simulink model "gm_inc_enc_v26_vnl"  (R2023a)
settings: Solver=FixedStepDiscrete  StartTime=0.0  StopTime=SimulationsDauer  RelTol=1e-3
undefined symbols (not defined in the file or in its folder): CW_CCW_Switch, d_axis_hit_CompareValue, DiscIntNeverNeededParam, f_ISR, IncPerTurn, inital_zero_speed_timeout, n_max, Offset_Position_elec, Offset_Position_mech, OmegaPerOverSampl, Periode, Phase_Delay_A, Phase_Delay_B, PolePair, QuadratureFactor, reciprocal_iterations, T_fpga, T_mech
libraries: simulink x25, hdlmdlgenlib x16, hdlsllib x4, dspsrcs4 x3, dspswit3 x2, spsEdgeDetectorLib x2, simulink_extras x1
(part 2 of 5)

== system gm_inc_enc_v26_vnl/Compare/Assert_count ==
  cosim : Inport
  dut : Inport  Port=2
  AssertEq : Assertion  StopWhenAssertionFail=off
  Compare To Zero : simulink/Logic and Bit Operations/Compare To Zero  relop===  OutDataTypeStr=boolean
  Relational Operator : RelationalOperator  Operator===  OutDataTypeStr=boolean  InputSameDT=off
  compare: count : Scope  NumInputPorts=3
  wires:
  Compare To Zero/1 -> compare: count/3  "err"
  Relational Operator/1 -> Compare To Zero/1, AssertEq/1
  cosim/1 -> compare: count/1, Relational Operator/1  "cosim"
  dut/1 -> compare: count/2, Relational Operator/2  "dut ref"

== system gm_inc_enc_v26_vnl/Compare/Assert_countPerPeriod_AXI4 ==
  cosim : Inport
  dut : Inport  Port=2
  AssertEq : Assertion  StopWhenAssertionFail=off
  Compare To Zero : simulink/Logic and Bit Operations/Compare To Zero  relop===  OutDataTypeStr=boolean
  Relational Operator : RelationalOperator  Operator===  OutDataTypeStr=boolean  InputSameDT=off
  compare: countPerPeriod_AXI4 : Scope  NumInputPorts=3
  wires:
  Compare To Zero/1 -> compare: countPerPeriod_AXI4/3  "err"
  Relational Operator/1 -> Compare To Zero/1, AssertEq/1
  cosim/1 -> compare: countPerPeriod_AXI4/1, Relational Operator/1  "cosim"
  dut/1 -> compare: countPerPeriod_AXI4/2, Relational Operator/2  "dut ref"

== system gm_inc_enc_v26_vnl/Compare/Assert_d-Axis-Hit ==
  cosim : Inport
  dut : Inport  Port=2
  AssertEq : Assertion  StopWhenAssertionFail=off
  Compare To Zero : simulink/Logic and Bit Operations/Compare To Zero  relop===  OutDataTypeStr=boolean
  Relational Operator : RelationalOperator  Operator===  OutDataTypeStr=boolean  InputSameDT=off
  compare: d-Axis-Hit : Scope  NumInputPorts=3
  wires:
  Compare To Zero/1 -> compare: d-Axis-Hit/3  "err"
  Relational Operator/1 -> Compare To Zero/1, AssertEq/1
  cosim/1 -> compare: d-Axis-Hit/1, Relational Operator/1  "cosim"
  dut/1 -> compare: d-Axis-Hit/2, Relational Operator/2  "dut ref"

== system gm_inc_enc_v26_vnl/Compare/Assert_d-Axis-Hit_WithCompare ==
  cosim : Inport
  dut : Inport  Port=2
  AssertEq : Assertion  StopWhenAssertionFail=off
  Compare To Zero : simulink/Logic and Bit Operations/Compare To Zero  relop===  OutDataTypeStr=boolean
  Relational Operator : RelationalOperator  Operator===  OutDataTypeStr=boolean  InputSameDT=off
  compare: d-Axis-Hit_WithCompare : Scope  NumInputPorts=3
  wires:
  Compare To Zero/1 -> compare: d-Axis-Hit_WithCompare/3  "err"
  Relational Operator/1 -> Compare To Zero/1, AssertEq/1
  cosim/1 -> compare: d-Axis-Hit_WithCompare/1, Relational Operator/1  "cosim"
  dut/1 -> compare: d-Axis-Hit_WithCompare/2, Relational Operator/2  "dut ref"

== system gm_inc_enc_v26_vnl/Compare/Assert_direction_AXI4 ==
  cosim : Inport
  dut : Inport  Port=2
  AssertEq : Assertion  StopWhenAssertionFail=off
  Compare To Zero : simulink/Logic and Bit Operations/Compare To Zero  relop===  OutDataTypeStr=boolean
  Relational Operator : RelationalOperator  Operator===  OutDataTypeStr=boolean  InputSameDT=off
  compare: direction_AXI4 : Scope  NumInputPorts=3
  wires:
  Compare To Zero/1 -> compare: direction_AXI4/3  "err"
  Relational Operator/1 -> Compare To Zero/1, AssertEq/1
  cosim/1 -> compare: direction_AXI4/1, Relational Operator/1  "cosim"
  dut/1 -> compare: direction_AXI4/2, Relational Operator/2  "dut ref"

== system gm_inc_enc_v26_vnl/Compare/Assert_edge ==
  cosim : Inport
  dut : Inport  Port=2
  AssertEq : Assertion  StopWhenAssertionFail=off
  Compare To Zero : simulink/Logic and Bit Operations/Compare To Zero  relop===  OutDataTypeStr=boolean
  Relational Operator : RelationalOperator  Operator===  OutDataTypeStr=boolean  InputSameDT=off
  compare: edge : Scope  NumInputPorts=3
  wires:
  Compare To Zero/1 -> compare: edge/3  "err"
  Relational Operator/1 -> Compare To Zero/1, AssertEq/1
  cosim/1 -> compare: edge/1, Relational Operator/1  "cosim"
  dut/1 -> compare: edge/2, Relational Operator/2  "dut ref"

== system gm_inc_enc_v26_vnl/Compare/Assert_new_measurement ==
  cosim : Inport
  dut : Inport  Port=2
  AssertEq : Assertion  StopWhenAssertionFail=off
  Compare To Zero : simulink/Logic and Bit Operations/Compare To Zero  relop===  OutDataTypeStr=boolean
  Relational Operator : RelationalOperator  Operator===  OutDataTypeStr=boolean  InputSameDT=off
  compare: new_measurement : Scope  NumInputPorts=3
  wires:
  Compare To Zero/1 -> compare: new_measurement/3  "err"
  Relational Operator/1 -> Compare To Zero/1, AssertEq/1
  cosim/1 -> compare: new_measurement/1, Relational Operator/1  "cosim"
  dut/1 -> compare: new_measurement/2, Relational Operator/2  "dut ref"

== system gm_inc_enc_v26_vnl/Compare/Assert_omega ==
  cosim : Inport
  dut : Inport  Port=2
  AssertEq : Assertion  StopWhenAssertionFail=off
  Compare To Zero : simulink/Logic and Bit Operations/Compare To Zero  relop===  OutDataTypeStr=boolean
  Relational Operator : RelationalOperator  Operator===  OutDataTypeStr=boolean  InputSameDT=off
  compare: omega : Scope  NumInputPorts=3
  wires:
  Compare To Zero/1 -> compare: omega/3  "err"
  Relational Operator/1 -> Compare To Zero/1, AssertEq/1
  cosim/1 -> compare: omega/1, Relational Operator/1  "cosim"
  dut/1 -> compare: omega/2, Relational Operator/2  "dut ref"

== system gm_inc_enc_v26_vnl/Compare/Assert_omegaA ==
  cosim : Inport
  dut : Inport  Port=2
  AssertEq : Assertion  StopWhenAssertionFail=off
  Compare To Zero : simulink/Logic and Bit Operations/Compare To Zero  relop===  OutDataTypeStr=boolean
  Relational Operator : RelationalOperator  Operator===  OutDataTypeStr=boolean  InputSameDT=off
  compare: omegaA : Scope  NumInputPorts=3
  wires:
  Compare To Zero/1 -> compare: omegaA/3  "err"
  Relational Operator/1 -> Compare To Zero/1, AssertEq/1
  cosim/1 -> compare: omegaA/1, Relational Operator/1  "cosim"
  dut/1 -> compare: omegaA/2, Relational Operator/2  "dut ref"

== system gm_inc_enc_v26_vnl/Compare/Assert_omegaB ==
  cosim : Inport
  dut : Inport  Port=2
  AssertEq : Assertion  StopWhenAssertionFail=off
  Compare To Zero : simulink/Logic and Bit Operations/Compare To Zero  relop===  OutDataTypeStr=boolean
  Relational Operator : RelationalOperator  Operator===  OutDataTypeStr=boolean  InputSameDT=off
  compare: omegaB : Scope  NumInputPorts=3
  wires:
  Compare To Zero/1 -> compare: omegaB/3  "err"
  Relational Operator/1 -> Compare To Zero/1, AssertEq/1
  cosim/1 -> compare: omegaB/1, Relational Operator/1  "cosim"
  dut/1 -> compare: omegaB/2, Relational Operator/2  "dut ref"

== system gm_inc_enc_v26_vnl/Compare/Assert_omegaNOTA ==
  cosim : Inport
  dut : Inport  Port=2
  AssertEq : Assertion  StopWhenAssertionFail=off
  Compare To Zero : simulink/Logic and Bit Operations/Compare To Zero  relop===  OutDataTypeStr=boolean
  Relational Operator : RelationalOperator  Operator===  OutDataTypeStr=boolean  InputSameDT=off
  compare: omegaNOTA : Scope  NumInputPorts=3
  wires:
  Compare To Zero/1 -> compare: omegaNOTA/3  "err"
  Relational Operator/1 -> Compare To Zero/1, AssertEq/1
  cosim/1 -> compare: omegaNOTA/1, Relational Operator/1  "cosim"
  dut/1 -> compare: omegaNOTA/2, Relational Operator/2  "dut ref"

== system gm_inc_enc_v26_vnl/Compare/Assert_omegaNOTB ==
  cosim : Inport
  dut : Inport  Port=2
  AssertEq : Assertion  StopWhenAssertionFail=off
  Compare To Zero : simulink/Logic and Bit Operations/Compare To Zero  relop===  OutDataTypeStr=boolean
  Relational Operator : RelationalOperator  Operator===  OutDataTypeStr=boolean  InputSameDT=off
  compare: omegaNOTB : Scope  NumInputPorts=3
  wires:
  Compare To Zero/1 -> compare: omegaNOTB/3  "err"
  Relational Operator/1 -> Compare To Zero/1, AssertEq/1
  cosim/1 -> compare: omegaNOTB/1, Relational Operator/1  "cosim"
  dut/1 -> compare: omegaNOTB/2, Relational Operator/2  "dut ref"

== system gm_inc_enc_v26_vnl/Compare/Assert_omega_AXI4 ==
  cosim : Inport
  dut : Inport  Port=2
  AssertEq : Assertion  StopWhenAssertionFail=off
  Compare To Zero : simulink/Logic and Bit Operations/Compare To Zero  relop===  OutDataTypeStr=boolean
  Relational Operator : RelationalOperator  Operator===  OutDataTypeStr=boolean  InputSameDT=off
  compare: omega_AXI4 : Scope  NumInputPorts=3
  wires:
  Compare To Zero/1 -> compare: omega_AXI4/3  "err"
  Relational Operator/1 -> Compare To Zero/1, AssertEq/1
  cosim/1 -> compare: omega_AXI4/1, Relational Operator/1  "cosim"
  dut/1 -> compare: omega_AXI4/2, Relational Operator/2  "dut ref"

== system gm_inc_enc_v26_vnl/Compare/Assert_omega_MA_N4 ==
  cosim : Inport
  dut : Inport  Port=2
  AssertEq : Assertion  StopWhenAssertionFail=off
  Compare To Zero : simulink/Logic and Bit Operations/Compare To Zero  relop===  OutDataTypeStr=boolean
  Relational Operator : RelationalOperator  Operator===  OutDataTypeStr=boolean  InputSameDT=off
  compare: omega_MA_N4 : Scope  NumInputPorts=3
  wires:
  Compare To Zero/1 -> compare: omega_MA_N4/3  "err"
  Relational Operator/1 -> Compare To Zero/1, AssertEq/1
  cosim/1 -> compare: omega_MA_N4/1, Relational Operator/1  "cosim"
  dut/1 -> compare: omega_MA_N4/2, Relational Operator/2  "dut ref"

== system gm_inc_enc_v26_vnl/Compare/Assert_omega_MA_N4_AXI ==
  cosim : Inport
  dut : Inport  Port=2
  AssertEq : Assertion  StopWhenAssertionFail=off
  Compare To Zero : simulink/Logic and Bit Operations/Compare To Zero  relop===  OutDataTypeStr=boolean
  Relational Operator : RelationalOperator  Operator===  OutDataTypeStr=boolean  InputSameDT=off
  compare: omega_MA_N4_AXI : Scope  NumInputPorts=3
  wires:
  Compare To Zero/1 -> compare: omega_MA_N4_AXI/3  "err"
  Relational Operator/1 -> Compare To Zero/1, AssertEq/1
  cosim/1 -> compare: omega_MA_N4_AXI/1, Relational Operator/1  "cosim"
  dut/1 -> compare: omega_MA_N4_AXI/2, Relational Operator/2  "dut ref"

== system gm_inc_enc_v26_vnl/Compare/Assert_position ==
  cosim : Inport
  dut : Inport  Port=2
  AssertEq : Assertion  StopWhenAssertionFail=off
  Compare To Zero : simulink/Logic and Bit Operations/Compare To Zero  relop===  OutDataTypeStr=boolean
  Relational Operator : RelationalOperator  Operator===  OutDataTypeStr=boolean  InputSameDT=off
  compare: position : Scope  NumInputPorts=3
  wires:
  Compare To Zero/1 -> compare: position/3  "err"
  Relational Operator/1 -> Compare To Zero/1, AssertEq/1
  cosim/1 -> compare: position/1, Relational Operator/1  "cosim"
  dut/1 -> compare: position/2, Relational Operator/2  "dut ref"

== system gm_inc_enc_v26_vnl/Compare/Assert_position_AXI4 ==
  cosim : Inport
  dut : Inport  Port=2
  AssertEq : Assertion  StopWhenAssertionFail=off
  Compare To Zero : simulink/Logic and Bit Operations/Compare To Zero  relop===  OutDataTypeStr=boolean
  Relational Operator : RelationalOperator  Operator===  OutDataTypeStr=boolean  InputSameDT=off
  compare: position_AXI4 : Scope  NumInputPorts=3
  wires:
  Compare To Zero/1 -> compare: position_AXI4/3  "err"
  Relational Operator/1 -> Compare To Zero/1, AssertEq/1
  cosim/1 -> compare: position_AXI4/1, Relational Operator/1  "cosim"
  dut/1 -> compare: position_AXI4/2, Relational Operator/2  "dut ref"

== system gm_inc_enc_v26_vnl/Compare/Assert_position_wOffset ==
  cosim : Inport
  dut : Inport  Port=2
  AssertEq : Assertion  StopWhenAssertionFail=off
  Compare To Zero : simulink/Logic and Bit Operations/Compare To Zero  relop===  OutDataTypeStr=boolean
  Relational Operator : RelationalOperator  Operator===  OutDataTypeStr=boolean  InputSameDT=off
  compare: position_wOffset : Scope  NumInputPorts=3
  wires:
  Compare To Zero/1 -> compare: position_wOffset/3  "err"
  Relational Operator/1 -> Compare To Zero/1, AssertEq/1
  cosim/1 -> compare: position_wOffset/1, Relational Operator/1  "cosim"
  dut/1 -> compare: position_wOffset/2, Relational Operator/2  "dut ref"

== system gm_inc_enc_v26_vnl/Compare/Assert_position_wOffset_AXI4 ==
  cosim : Inport
  dut : Inport  Port=2
  AssertEq : Assertion  StopWhenAssertionFail=off
  Compare To Zero : simulink/Logic and Bit Operations/Compare To Zero  relop===  OutDataTypeStr=boolean
  Relational Operator : RelationalOperator  Operator===  OutDataTypeStr=boolean  InputSameDT=off
  compare: position_wOffset_AXI4 : Scope  NumInputPorts=3
  wires:
  Compare To Zero/1 -> compare: position_wOffset_AXI4/3  "err"
  Relational Operator/1 -> Compare To Zero/1, AssertEq/1
  cosim/1 -> compare: position_wOffset_AXI4/1, Relational Operator/1  "cosim"
  dut/1 -> compare: position_wOffset_AXI4/2, Relational Operator/2  "dut ref"

== system gm_inc_enc_v26_vnl/Compare/Assert_theta_el ==
  cosim : Inport
  dut : Inport  Port=2
  AssertEq : Assertion  StopWhenAssertionFail=off
  Compare To Zero : simulink/Logic and Bit Operations/Compare To Zero  relop===  OutDataTypeStr=boolean
  Relational Operator : RelationalOperator  Operator===  OutDataTypeStr=boolean  InputSameDT=off
  compare: theta_el : Scope  NumInputPorts=3
  wires:
  Compare To Zero/1 -> compare: theta_el/3  "err"
  Relational Operator/1 -> Compare To Zero/1, AssertEq/1
  cosim/1 -> compare: theta_el/1, Relational Operator/1  "cosim"
  dut/1 -> compare: theta_el/2, Relational Operator/2  "dut ref"

== system gm_inc_enc_v26_vnl/Compare/Assert_theta_el_AXI4 ==
  cosim : Inport
  dut : Inport  Port=2
  AssertEq : Assertion  StopWhenAssertionFail=off
  Compare To Zero : simulink/Logic and Bit Operations/Compare To Zero  relop===  OutDataTypeStr=boolean
  Relational Operator : RelationalOperator  Operator===  OutDataTypeStr=boolean  InputSameDT=off
  compare: theta_el_AXI4 : Scope  NumInputPorts=3
  wires:
  Compare To Zero/1 -> compare: theta_el_AXI4/3  "err"
  Relational Operator/1 -> Compare To Zero/1, AssertEq/1
  cosim/1 -> compare: theta_el_AXI4/1, Relational Operator/1  "cosim"
  dut/1 -> compare: theta_el_AXI4/2, Relational Operator/2  "dut ref"

== system gm_inc_enc_v26_vnl/Compare/Assert_timeout_active ==
  cosim : Inport
  dut : Inport  Port=2
  AssertEq : Assertion  StopWhenAssertionFail=off
  Compare To Zero : simulink/Logic and Bit Operations/Compare To Zero  relop===  OutDataTypeStr=boolean
  Relational Operator : RelationalOperator  Operator===  OutDataTypeStr=boolean  InputSameDT=off
  compare: timeout_active : Scope  NumInputPorts=3
  wires:
  Compare To Zero/1 -> compare: timeout_active/3  "err"
  Relational Operator/1 -> Compare To Zero/1, AssertEq/1
  cosim/1 -> compare: timeout_active/1, Relational Operator/1  "cosim"
  dut/1 -> compare: timeout_active/2, Relational Operator/2  "dut ref"

== system gm_inc_enc_v26_vnl/Compare/CleanupScopes ==

== system gm_inc_enc_v26_vnl/Compare/Enable ==

== system gm_inc_enc_v26_vnl/Create_Referenz/IncrementalEncoder_Floating ==
  A : Inport
  B : Inport  Port=2
  I : Inport  Port=3
  poles : Inport  Port=4
  Add : Sum  Inputs=+-  OutDataTypeStr=fixdt(1,16,0)
  Counter3 : dspswit3/Counter  Direction=Up  CountEvent=Either edge  CounterSize=User defined  MaxCount=IncPerTurn*4  InitialCount=0  Output=Count  HitValue=32  ResetInput=on  SamplesPerFrame=1  Ts=1  CntDtype=double  HitDtype=Logical
  CutTheta_0_2PI : Subsystem
  Edge Detector2 : spsEdgeDetectorLib/Edge Detector  model=Rising  ic=0  Ts=-1
  Edge Detector3 : spsEdgeDetectorLib/Edge Detector  model=Rising  ic=0  Ts=-1
  Logical Operator1 : Logic  Operator=XOR  AllPortsSameDT=off  OutDataTypeStr=boolean
  Logical Operator3 : Logic  AllPortsSameDT=off  OutDataTypeStr=boolean
  Logical Operator4 : Logic  Operator=NOT  AllPortsSameDT=off  OutDataTypeStr=boolean
  Logical Operator5 : Logic  AllPortsSameDT=off  OutDataTypeStr=boolean
  Logical Operator6 : Logic  Operator=NOT  AllPortsSameDT=off  OutDataTypeStr=boolean
  Product : Product
  S-R Flip-Flop1 : simulink_extras/Flip Flops/S-R Flip-Flop  initial_condition=0
  Scope1 : Scope  NumInputPorts=4
  cut_theta_2pi : Gain  Gain=(2*pi)/(IncPerTurn*QuadratureFactor)
  cut_theta_2pi1 : Gain  Gain=(2*pi)/(IncPerTurn*QuadratureFactor)
  n_aus_theta_v4 : Subsystem
  rpm : Outport  VectorParamsAs1DForOutWhenUnconnected=off
  theta_mech : Outport  Port=2  VectorParamsAs1DForOutWhenUnconnected=off
  theta_elec : Outport  Port=3  VectorParamsAs1DForOutWhenUnconnected=off
  direction : Outport  Port=4  VectorParamsAs1DForOutWhenUnconnected=off
  wires:
  I/1 -> Counter3/2
  Counter3/1 -> Product/1, cut_theta_2pi/1, Scope1/1
  n_aus_theta_v4/1(n) -> rpm/1
  Logical Operator1/1 -> Scope1/4, Counter3/1
  cut_theta_2pi/1 -> Scope1/2, n_aus_theta_v4/1(theta), theta_mech/1
  Product/1 -> cut_theta_2pi1/1
  poles/1 -> Product/2
  cut_theta_2pi1/1 -> CutTheta_0_2PI/1(In1)
  CutTheta_0_2PI/1(Out1) -> theta_elec/1
  Edge Detector2/1 -> Logical Operator3/1
  Logical Operator4/1 -> Logical Operator3/2
  Logical Operator3/1 -> S-R Flip-Flop1/1
  Edge Detector3/1 -> Logical Operator5/1
  Logical Operator6/1 -> Logical Operator5/2
  Logical Operator5/1 -> S-R Flip-Flop1/2
  S-R Flip-Flop1/1 -> Add/1
  S-R Flip-Flop1/2 -> Add/2
  A/1 -> Logical Operator6/1, Edge Detector2/1, Logical Operator1/1
  B/1 -> Edge Detector3/1, Logical Operator4/1, Logical Operator1/2
  Add/1 -> direction/1

== system gm_inc_enc_v26_vnl/Create_Referenz/n_aus_theta ==
  count : Inport
  T : Inport  Port=2
  1/rps->1/omega : Gain  Gain=1/(2*pi)  OutDataTypeStr=double
  Add : Sum  Inputs=+-
  Add1 : Sum
  Constant : Constant  Value=0  OutDataTypeStr=double  SampleTime=-1
  Constant1 : Constant  Value=0  OutDataTypeStr=double  SampleTime=-1
  Constant2 : Constant  Value=0  OutDataTypeStr=double  SampleTime=-1
  Divide1 : Product  Inputs=/
  ProtectOverflow_T_count : Switch  Threshold=50  SaturateOnIntegerOverflow=off  InputSameDT=off
  ProtectOverflow_rps : Switch  Threshold=50  OutDataTypeStr=double  SaturateOnIntegerOverflow=off  InputSameDT=off
  Scope1 : Scope  NumInputPorts=4
  Scope2 : Scope  NumInputPorts=4
  T_count : Delay  DelayLength=1
  T_count_switch : Switch  Criteria=u2 ~= 0  SaturateOnIntegerOverflow=off  InputSameDT=off
  count_old : Delay  DelayLength=1
  count_old_switch : Switch  Criteria=u2 ~= 0  SaturateOnIntegerOverflow=off  InputSameDT=off
  speed_old : Delay  DelayLength=1
  speed_old_switch : Switch  Criteria=u2 ~= 0  SaturateOnIntegerOverflow=off  InputSameDT=off
  rpm : Outport  VectorParamsAs1DForOutWhenUnconnected=off
  wires:
  count_old_switch/1 -> count_old/1
  count_old/1 -> count_old_switch/3, Add/2
  Constant/1 -> T_count_switch/1
  Add/1 -> speed_old_switch/2, count_old_switch/2, Scope1/1, T_count_switch/2
  Constant1/1 -> ProtectOverflow_T_count/1
  ProtectOverflow_rps/1 -> 1/rps->1/omega/1, Scope2/1
  Constant2/1 -> ProtectOverflow_rps/1
  speed_old_switch/1 -> ProtectOverflow_rps/3, Scope2/3, speed_old/1
  speed_old/1 -> speed_old_switch/3
  T/1 -> Scope2/4, Add1/1
  ProtectOverflow_T_count/1 -> T_count/1
  T_count/1 -> Scope1/4, Add1/2
  Add1/1 -> Scope2/2, speed_old_switch/1, T_count_switch/3
  count/1 -> Add/1, count_old_switch/1
  T_count_switch/1 -> ProtectOverflow_rps/2, Scope1/2, ProtectOverflow_T_count/2, ProtectOverflow_T_count/3
  1/rps->1/omega/1 -> Divide1/1
  Divide1/1 -> rpm/1

== system gm_inc_enc_v26_vnl/IncEnc_V26/AB-Line-Switch ==
  A_in : Inport  OutDataTypeStr=boolean  PortDimensions=1  SampleTime=1e-08
  B_in : Inport  Port=2  OutDataTypeStr=boolean  PortDimensions=1  SampleTime=1e-08
  CW_CCW_Switch : Inport  Port=3  OutDataTypeStr=boolean  PortDimensions=1  SampleTime=1e-08
  Switch : Switch  Criteria=u2 > Threshold  Threshold=double(0)  OutDataTypeStr=boolean  SampleTime=1e-08  SaturateOnIntegerOverflow=off  InputSameDT=off
  Switch1 : Switch  Criteria=u2 > Threshold  Threshold=double(0)  OutDataTypeStr=boolean  SampleTime=1e-08  SaturateOnIntegerOverflow=off  InputSameDT=off
  rd_0 : Delay  DelayLength=double(1)  InitialCondition=0  SampleTime=1e-08
  A_out : Outport  SampleTime=1e-08
  B_out : Outport  Port=2  SampleTime=1e-08
  wires:
  rd_0/1 -> Switch1/2, Switch/2
  CW_CCW_Switch/1 -> rd_0/1
  Switch1/1 -> B_out/1
  Switch/1 -> A_out/1
  B_in/1 -> Switch/1, Switch1/3
  A_in/1 -> Switch/3, Switch1/1

== system gm_inc_enc_v26_vnl/IncEnc_V26/Check d-Axis-Hit ==
  Count_in : Inport  OutDataTypeStr=uint16  PortDimensions=1  SampleTime=1e-08
  IncPerTurn_elek_AXI4 : Inport  Port=2  OutDataTypeStr=uint16  PortDimensions=1  SampleTime=1e-08
  Constant : Constant  Value=0  OutDataTypeStr=uint16  SampleTime=1e-08
  Equal : RelationalOperator  Operator===  OutDataTypeStr=boolean  SampleTime=1e-08  InputSameDT=off
  Equal1 : RelationalOperator  Operator===  OutDataTypeStr=boolean  SampleTime=1e-08  InputSameDT=off
  OR : Logic  Operator=OR  AllPortsSameDT=off  OutDataTypeStr=boolean  SampleTime=1e-08
  d-axis-hit : Outport  SampleTime=1e-08  VectorParamsAs1DForOutWhenUnconnected=off
  wires:
  OR/1 -> d-axis-hit/1
  Equal1/1 -> OR/2
  Equal/1 -> OR/1
  Constant/1 -> Equal/2
  IncPerTurn_elek_AXI4/1 -> Equal1/2
  Count_in/1 -> Equal/1, Equal1/1

== system gm_inc_enc_v26_vnl/IncEnc_V26/Check d-Axis-Hit_WithCompare ==
  Count_in : Inport  OutDataTypeStr=uint16  PortDimensions=1  SampleTime=1e-08
  Counter_Compare : Inport  Port=2  OutDataTypeStr=uint16  PortDimensions=1  SampleTime=1e-08
  Equal : RelationalOperator  Operator===  OutDataTypeStr=boolean  SampleTime=1e-08  InputSameDT=off
  d-axis-hit : Outport  SampleTime=1e-08  VectorParamsAs1DForOutWhenUnconnected=off
  wires:
  Equal/1 -> d-axis-hit/1
  Counter_Compare/1 -> Equal/2
  Count_in/1 -> Equal/1

== system gm_inc_enc_v26_vnl/IncEnc_V26/Counter ==
  note: 1 for one cycle if edge recognized
  note: Reset
  Enable_ctr : Inport  OutDataTypeStr=boolean  PortDimensions=1  SampleTime=1e-08
  I_line : Inport  Port=2  OutDataTypeStr=boolean  PortDimensions=1  SampleTime=1e-08
  Detec_edge : Sum  Inputs=+-  AccumDataTypeStr=int8  OutDataTypeStr=int8  SampleTime=1e-08
  Reset_flag : Sum  Inputs=+-  AccumDataTypeStr=uint8  OutDataTypeStr=uint8  SampleTime=1e-08
  rd_0 : Delay  DelayLength=double(1)  InitialCondition=0  SampleTime=1e-08
  rd_1 : Delay  DelayLength=double(1)  InitialCondition=0  SampleTime=1e-08
  rd_2 : Delay  DelayLength=double(1)  InitialCondition=0  SampleTime=1e-08
  reset_old_switch : Switch  Criteria=u2 ~= 0  Threshold=double(0)  OutDataTypeStr=boolean  SampleTime=1e-08  SaturateOnIntegerOverflow=off  InputSameDT=off
  reset_old_switch1 : Switch  Criteria=u2 ~= 0  Threshold=double(0)  OutDataTypeStr=boolean  SampleTime=1e-08  SaturateOnIntegerOverflow=off  InputSameDT=off
  Edge : Outport  SampleTime=1e-08  VectorParamsAs1DForOutWhenUnconnected=off
  Reset : Outport  Port=2  SampleTime=1e-08  VectorParamsAs1DForOutWhenUnconnected=off
  wires:
  rd_2/1 -> reset_old_switch/3, Reset_flag/2
  reset_old_switch/1 -> rd_2/1
  rd_1/1 -> reset_old_switch1/3, Detec_edge/2
  reset_old_switch1/1 -> rd_1/1
  rd_0/1 -> Detec_edge/1, reset_old_switch1/1
  Enable_ctr/1 -> rd_0/1
  Reset_flag/1 -> reset_old_switch/2, Reset/1
  Detec_edge/1 -> reset_old_switch1/2, Edge/1
  I_line/1 -> reset_old_switch/1, Reset_flag/1

== system gm_inc_enc_v26_vnl/IncEnc_V26/Counter_Theta_el_wOffset ==
  note: Check if count is to big 0-Increments
  note: Count
  note: Check if count is to small
  Edge : Inport  OutDataTypeStr=int8  PortDimensions=1  SampleTime=1e-08
  Reset : Inport  Port=2  OutDataTypeStr=uint8  PortDimensions=1  SampleTime=1e-08
  IncsPerTurn : Inport  Port=3  OutDataTypeStr=uint16  PortDimensions=1  SampleTime=1e-08
  Dir : Inport  Port=4  OutDataTypeStr=fixdt(1, 4, 0)  PortDimensions=1  SampleTime=1e-08
  Position_offset : Inport  Port=5  OutDataTypeStr=uint16  PortDimensions=1  SampleTime=1e-08
  Add1 : Sum  AccumDataTypeStr=int16  OutDataTypeStr=int16  SampleTime=1e-08
  Constant1 : Constant  Value=0  OutDataTypeStr=int16  SampleTime=1e-08
  Constant2 : Constant  OutDataTypeStr=int16  SampleTime=1e-08
  Constant3 : Constant  Value=0  OutDataTypeStr=int16  SampleTime=1e-08
  Constant5 : Constant  Value=-1  OutDataTypeStr=int16  SampleTime=1e-08
  Relational Operator : RelationalOperator  Operator=>  OutDataTypeStr=boolean  SampleTime=1e-08  InputSameDT=off
  Relational Operator1 : RelationalOperator  Operator=<=  OutDataTypeStr=boolean  SampleTime=1e-08  InputSameDT=off
  Resett_switch1 : Switch  Criteria=u2 ~= 0  Threshold=double(0)  OutDataTypeStr=uint16  SampleTime=1e-08  SaturateOnIntegerOverflow=off  InputSameDT=off
  Resett_switch2 : Switch  Criteria=u2 ~= 0  Threshold=double(0)  OutDataTypeStr=int16  SampleTime=1e-08  SaturateOnIntegerOverflow=off  InputSameDT=off
  Resett_switch3 : Switch  Criteria=u2 ~= 0  Threshold=double(0)  OutDataTypeStr=int16  SampleTime=1e-08  SaturateOnIntegerOverflow=off  InputSameDT=off
  only_use_for_neg_speed : Switch  Threshold=double(1)  OutDataTypeStr=int16  SampleTime=1e-08  SaturateOnIntegerOverflow=off  InputSameDT=off
  reset_old{1..7} (7 alike) : Delay  DelayLength=double(1)  InitialCondition=0  SampleTime=1e-08
  speed_old_switch1 : Switch  Criteria=u2 ~= 0  Threshold=double(0)  OutDataTypeStr=int16  SampleTime=1e-08  SaturateOnIntegerOverflow=off  InputSameDT=off
  speed_old_switch2 : Switch  Threshold=double(1)  OutDataTypeStr=int16  SampleTime=1e-08  SaturateOnIntegerOverflow=off  InputSameDT=off
  count : Outport  SampleTime=1e-08  VectorParamsAs1DForOutWhenUnconnected=off
  wires:
  reset_old3/1 -> Resett_switch1/2
  Relational Operator/1 -> reset_old3/1
  Resett_switch3/1 -> Relational Operator1/1, Resett_switch1/3
  only_use_for_neg_speed/1 -> Resett_switch3/2
  reset_old2/1 -> only_use_for_neg_speed/3
  Relational Operator1/1 -> reset_old2/1
  reset_old1/1 -> Add1/2
  Add1/1 -> Resett_switch2/3
  Resett_switch2/1 -> Resett_switch3/3
  speed_old_switch2/1 -> reset_old4/1
  speed_old_switch1/1 -> Add1/1
  reset_old7/1 -> Resett_switch2/1
  reset_old6/1 -> only_use_for_neg_speed/2, speed_old_switch2/2
  reset_old5/1 -> Relational Operator/2, Resett_switch3/1
  reset_old4/1 -> speed_old_switch1/1
  Resett_switch1/1 -> reset_old1/1, Relational Operator/1, count/1
  Constant5/1 -> speed_old_switch2/3
  Constant3/1 -> speed_old_switch1/3
  Constant2/1 -> speed_old_switch2/1
  Constant1/1 -> Relational Operator1/2, Resett_switch1/1, only_use_for_neg_speed/1
  Position_offset/1 -> reset_old7/1
  Dir/1 -> reset_old6/1
  IncsPerTurn/1 -> reset_old5/1
  Reset/1 -> Resett_switch2/2
  Edge/1 -> speed_old_switch1/2

== system gm_inc_enc_v26_vnl/IncEnc_V26/Counter_position ==
  note: Count
  note: Check if count is to big 0-Increments
  note: Check if count is to small
  Edge : Inport  OutDataTypeStr=int8  PortDimensions=1  SampleTime=1e-08
  Reset : Inport  Port=2  OutDataTypeStr=uint8  PortDimensions=1  SampleTime=1e-08
  IncsPerTurn : Inport  Port=3  OutDataTypeStr=uint16  PortDimensions=1  SampleTime=1e-08
  Dir : Inport  Port=4  OutDataTypeStr=fixdt(1, 4, 0)  PortDimensions=1  SampleTime=1e-08
  Add1 : Sum  AccumDataTypeStr=int16  OutDataTypeStr=int16  SampleTime=1e-08
  Constant1 : Constant  Value=0  OutDataTypeStr=int16  SampleTime=1e-08
  Constant2 : Constant  OutDataTypeStr=int16  SampleTime=1e-08
  Constant3 : Constant  Value=0  OutDataTypeStr=int16  SampleTime=1e-08
  Constant4 : Constant  Value=0  OutDataTypeStr=int16  SampleTime=1e-08
  Constant5 : Constant  Value=-1  OutDataTypeStr=int16  SampleTime=1e-08
  Relational Operator : RelationalOperator  Operator=>  OutDataTypeStr=boolean  SampleTime=1e-08  InputSameDT=off
  Relational Operator1 : RelationalOperator  Operator=<=  OutDataTypeStr=boolean  SampleTime=1e-08  InputSameDT=off
  Resett_switch1 : Switch  Criteria=u2 ~= 0  Threshold=double(0)  OutDataTypeStr=uint16  SampleTime=1e-08  SaturateOnIntegerOverflow=off  InputSameDT=off
  Resett_switch2 : Switch  Criteria=u2 ~= 0  Threshold=double(0)  OutDataTypeStr=int16  SampleTime=1e-08  SaturateOnIntegerOverflow=off  InputSameDT=off
  Resett_switch3 : Switch  Criteria=u2 ~= 0  Threshold=double(0)  OutDataTypeStr=int16  SampleTime=1e-08  SaturateOnIntegerOverflow=off  InputSameDT=off
  only_use_for_neg_speed : Switch  Threshold=double(1)  OutDataTypeStr=int16  SampleTime=1e-08  SaturateOnIntegerOverflow=off  InputSameDT=off
  rd_0 : Delay  DelayLength=double(2)  InitialCondition=0  SampleTime=1e-08
  rd_{1,3..5} (4 alike) : Delay  DelayLength=double(1)  InitialCondition=0  SampleTime=1e-08
  rd_2 : Delay  DelayLength=double(3)  InitialCondition=0  SampleTime=1e-08
  speed_old_switch1 : Switch  Criteria=u2 ~= 0  Threshold=double(0)  OutDataTypeStr=int16  SampleTime=1e-08  SaturateOnIntegerOverflow=off  InputSameDT=off
  speed_old_switch2 : Switch  Threshold=double(1)  OutDataTypeStr=int16  SampleTime=1e-08  SaturateOnIntegerOverflow=off  InputSameDT=off
  count : Outport  SampleTime=1e-08  VectorParamsAs1DForOutWhenUnconnected=off
  wires:
  rd_5/1 -> Relational Operator/1, Add1/2
  Resett_switch1/1 -> rd_5/1, count/1
  rd_2/1 -> speed_old_switch2/2, only_use_for_neg_speed/2
  Dir/1 -> rd_2/1
  rd_1/1 -> Relational Operator/2
  rd_0/1 -> rd_1/1, Resett_switch3/1
  IncsPerTurn/1 -> rd_0/1
  rd_3/1 -> speed_old_switch1/1
  rd_4/1 -> only_use_for_neg_speed/3
  Relational Operator/1 -> Resett_switch1/2
  Resett_switch3/1 -> Relational Operator1/1, Resett_switch1/3
  only_use_for_neg_speed/1 -> Resett_switch3/2
  Relational Operator1/1 -> rd_4/1
  Add1/1 -> Resett_switch2/3
  Resett_switch2/1 -> Resett_switch3/3
  speed_old_switch2/1 -> rd_3/1
  speed_old_switch1/1 -> Add1/1
  Constant5/1 -> speed_old_switch2/3
  Constant4/1 -> only_use_for_neg_speed/1, Resett_switch1/1, Relational Operator1/2
  Constant3/1 -> speed_old_switch1/3
  Constant2/1 -> speed_old_switch2/1
  Constant1/1 -> Resett_switch2/1
  Reset/1 -> Resett_switch2/2
  Edge/1 -> speed_old_switch1/2

== system gm_inc_enc_v26_vnl/IncEnc_V26/Counter_position_wOffset ==
  note: Check if count is to small
  note: Count
  note: Check if count is to big 0-Increments
  Edge : Inport  OutDataTypeStr=int8  PortDimensions=1  SampleTime=1e-08
  Reset : Inport  Port=2  OutDataTypeStr=uint8  PortDimensions=1  SampleTime=1e-08
  IncsPerTurn : Inport  Port=3  OutDataTypeStr=uint16  PortDimensions=1  SampleTime=1e-08
  Dir : Inport  Port=4  OutDataTypeStr=fixdt(1, 4, 0)  PortDimensions=1  SampleTime=1e-08
  Position_offset : Inport  Port=5  OutDataTypeStr=uint16  PortDimensions=1  SampleTime=1e-08
  Add1 : Sum  AccumDataTypeStr=int16  OutDataTypeStr=int16  SampleTime=1e-08
  Constant1 : Constant  Value=0  OutDataTypeStr=int16  SampleTime=1e-08
  Constant2 : Constant  OutDataTypeStr=int16  SampleTime=1e-08
  Constant3 : Constant  Value=0  OutDataTypeStr=int16  SampleTime=1e-08
  Constant5 : Constant  Value=-1  OutDataTypeStr=int16  SampleTime=1e-08
  Relational Operator : RelationalOperator  Operator=>  OutDataTypeStr=boolean  SampleTime=1e-08  InputSameDT=off
  Relational Operator1 : RelationalOperator  Operator=<=  OutDataTypeStr=boolean  SampleTime=1e-08  InputSameDT=off
  Resett_switch1 : Switch  Criteria=u2 ~= 0  Threshold=double(0)  OutDataTypeStr=uint16  SampleTime=1e-08  SaturateOnIntegerOverflow=off  InputSameDT=off
  Resett_switch2 : Switch  Criteria=u2 ~= 0  Threshold=double(0)  OutDataTypeStr=int16  SampleTime=1e-08  SaturateOnIntegerOverflow=off  InputSameDT=off
  Resett_switch3 : Switch  Criteria=u2 ~= 0  Threshold=double(0)  OutDataTypeStr=int16  SampleTime=1e-08  SaturateOnIntegerOverflow=off  InputSameDT=off
  only_use_for_neg_speed : Switch  Threshold=double(1)  OutDataTypeStr=int16  SampleTime=1e-08  SaturateOnIntegerOverflow=off  InputSameDT=off
  reset_old{1..7} (7 alike) : Delay  DelayLength=double(1)  InitialCondition=0  SampleTime=1e-08
  speed_old_switch1 : Switch  Criteria=u2 ~= 0  Threshold=double(0)  OutDataTypeStr=int16  SampleTime=1e-08  SaturateOnIntegerOverflow=off  InputSameDT=off
  speed_old_switch2 : Switch  Threshold=double(1)  OutDataTypeStr=int16  SampleTime=1e-08  SaturateOnIntegerOverflow=off  InputSameDT=off
  count : Outport  SampleTime=1e-08  VectorParamsAs1DForOutWhenUnconnected=off
  wires:
  Edge/1 -> speed_old_switch1/2
  Reset/1 -> Resett_switch2/2
  IncsPerTurn/1 -> reset_old5/1
  Dir/1 -> reset_old6/1
  Position_offset/1 -> reset_old7/1
  Constant1/1 -> only_use_for_neg_speed/1, Resett_switch1/1, Relational Operator1/2
  Constant2/1 -> speed_old_switch2/1
  Constant3/1 -> speed_old_switch1/3
  Constant5/1 -> speed_old_switch2/3
  Resett_switch1/1 -> count/1, Relational Operator/1, reset_old1/1
  reset_old4/1 -> speed_old_switch1/1
  reset_old5/1 -> Resett_switch3/1, Relational Operator/2
  reset_old6/1 -> speed_old_switch2/2, only_use_for_neg_speed/2
  reset_old7/1 -> Resett_switch2/1
  speed_old_switch1/1 -> Add1/1
  speed_old_switch2/1 -> reset_old4/1
  Resett_switch2/1 -> Resett_switch3/3
  Add1/1 -> Resett_switch2/3
  reset_old1/1 -> Add1/2
  Relational Operator1/1 -> reset_old2/1
  reset_old2/1 -> only_use_for_neg_speed/3
  only_use_for_neg_speed/1 -> Resett_switch3/2
  Resett_switch3/1 -> Resett_switch1/3, Relational Operator1/1
  Relational Operator/1 -> reset_old3/1
  reset_old3/1 -> Resett_switch1/2

== system gm_inc_enc_v26_vnl/IncEnc_V26/Direction ==
  A : Inport  OutDataTypeStr=boolean  PortDimensions=1  SampleTime=1e-08
  B : Inport  Port=2  OutDataTypeStr=boolean  PortDimensions=1  SampleTime=1e-08
  Add : Sum  Inputs=+-  AccumDataTypeStr=fixdt(1, 4, 0)  OutDataTypeStr=fixdt(1, 4, 0)  SampleTime=1e-08
  Add1 : Sum  Inputs=+-  AccumDataTypeStr=fixdt(1, 4, 0)  OutDataTypeStr=fixdt(1, 4, 0)  SampleTime=1e-08
  Add2 : Sum  AccumDataTypeStr=fixdt(1, 4, 0)  OutDataTypeStr=fixdt(1, 4, 0)  SampleTime=1e-08
  Change : Sum  AccumDataTypeStr=fixdt(1, 4, 0)  OutDataTypeStr=fixdt(1, 4, 0)  SampleTime=1e-08
  Save_Direction : Switch  Criteria=u2 ~= 0  Threshold=double(0)  OutDataTypeStr=fixdt(1, 4, 0)  SampleTime=1e-08  SaturateOnIntegerOverflow=off  InputSameDT=off
  T_count_switch : Switch  Threshold=double(1)  OutDataTypeStr=fixdt(1, 4, 0)  SampleTime=1e-08  SaturateOnIntegerOverflow=off  InputSameDT=off
  TrnLeft : Sum  Inputs=+-  AccumDataTypeStr=fixdt(1, 4, 0)  OutDataTypeStr=fixdt(1, 4, 0)  SampleTime=1e-08
  TrnRight : Sum  Inputs=+-  AccumDataTypeStr=fixdt(1, 4, 0)  OutDataTypeStr=fixdt(1, 4, 0)  SampleTime=1e-08
  TurnLeft : Constant  Value=-1  OutDataTypeStr=fixdt(1, 4, 0)  SampleTime=1e-08
  TurnRight : Constant  OutDataTypeStr=fixdt(1, 4, 0)  SampleTime=1e-08
  count_old_switch : Switch  Criteria=u2 ~= 0  Threshold=double(0)  OutDataTypeStr=boolean  SampleTime=1e-08  SaturateOnIntegerOverflow=off  InputSameDT=off
  count_old_switch1 : Switch  Criteria=u2 ~= 0  Threshold=double(0)  OutDataTypeStr=boolean  SampleTime=1e-08  SaturateOnIntegerOverflow=off  InputSameDT=off
  nothing : Constant  Value=0  OutDataTypeStr=fixdt(1, 4, 0)  SampleTime=1e-08
  nothing1 : Constant  Value=0  OutDataTypeStr=fixdt(1, 4, 0)  SampleTime=1e-08
  rd_{0..8} (9 alike) : Delay  DelayLength=double(1)  InitialCondition=0  SampleTime=1e-08
  speed_old_switch : Switch  Threshold=double(1)  OutDataTypeStr=fixdt(1, 4, 0)  SampleTime=1e-08  SaturateOnIntegerOverflow=off  InputSameDT=off
  t : hdlmdlgenlib/Buffer
  t1 : hdlmdlgenlib/Buffer
  Dir : Outport  SampleTime=1e-08  VectorParamsAs1DForOutWhenUnconnected=off
  wires:
  rd_7/1 -> TrnLeft/1, count_old_switch1/2
  Add1/1 -> rd_7/1
  rd_3/1 -> TrnRight/1, count_old_switch/2
  Add/1 -> rd_3/1
  rd_4/1 -> count_old_switch1/1, TrnRight/2
  B/1 -> rd_4/1, Add1/1
  rd_1/1 -> TrnLeft/2, count_old_switch/1
  A/1 -> rd_1/1, Add/1
  rd_6/1 -> count_old_switch1/3
  rd_8/1 -> Save_Direction/3
  rd_2/1 -> count_old_switch/3
  rd_0/1 -> T_count_switch/1
  rd_5/1 -> speed_old_switch/1
  Save_Direction/1 -> t1/1
  count_old_switch1/1 -> Add1/2, rd_6/1
  count_old_switch/1 -> Add/2, rd_2/1
  speed_old_switch/1 -> Add2/2, Change/2
  nothing1/1 -> T_count_switch/3
  nothing/1 -> speed_old_switch/3
  t1/1 -> Dir/1, rd_8/1
  TurnRight/1 -> rd_0/1
  TurnLeft/1 -> rd_5/1
  TrnRight/1 -> T_count_switch/2
  TrnLeft/1 -> speed_old_switch/2
  T_count_switch/1 -> Add2/1, Change/1
  t/1 -> Save_Direction/2
  Change/1 -> t/1
  Add2/1 -> Save_Direction/1

== system gm_inc_enc_v26_vnl/IncEnc_V26/Index_Latch ==
  Reset_in : Inport  OutDataTypeStr=uint8  PortDimensions=1  SampleTime=1e-08
  Constant : Constant  OutDataTypeStr=boolean  SampleTime=1e-08
  Constant4 : Constant  Value=0  OutDataTypeStr=boolean  SampleTime=1e-08
  OR : Logic  Operator=OR  AllPortsSameDT=off  OutDataTypeStr=boolean  SampleTime=1e-08
  Switch : Switch  Criteria=u2 > Threshold  Threshold=double(0)  OutDataTypeStr=boolean  SampleTime=1e-08  SaturateOnIntegerOverflow=off  InputSameDT=off
  rd_0 : Delay  DelayLength=double(1)  InitialCondition=0  SampleTime=1e-08
  Index_found : Outport  SampleTime=1e-08
  wires:
  rd_0/1 -> OR/2
  OR/1 -> Switch/2
  Switch/1 -> Index_found/1, rd_0/1
  Constant4/1 -> Switch/3
  Constant/1 -> Switch/1
  Reset_in/1 -> OR/1

== system gm_inc_enc_v26_vnl/IncEnc_V26/count_lines ==
  note: Set new counter value
  note: Check if count is to big in order to safe for value overflow
  note: Count
  Edge : Inport  OutDataTypeStr=int8  PortDimensions=1  SampleTime=1e-08
  Reset : Inport  Port=2  OutDataTypeStr=boolean  PortDimensions=1  SampleTime=1e-08
  IncsPerTurn : Inport  Port=3  OutDataTypeStr=uint16  PortDimensions=1  SampleTime=1e-08
  Add1 : Sum  AccumDataTypeStr=int16  OutDataTypeStr=int16  SampleTime=1e-08
  Constant1 : Constant  Value=0  OutDataTypeStr=int16  SampleTime=1e-08
  Constant2 : Constant  OutDataTypeStr=int16  SampleTime=1e-08
  Constant3 : Constant  Value=0  OutDataTypeStr=int16  SampleTime=1e-08
  Constant4 : Constant  Value=10  OutDataTypeStr=int16  SampleTime=1e-08
  Relational Operator : RelationalOperator  Operator=>  OutDataTypeStr=boolean  SampleTime=1e-08  InputSameDT=off
  Reset_when_overflow : Sum  AccumDataTypeStr=fixdt(1, 18, 0)  OutDataTypeStr=int16  SampleTime=1e-08
  Resett_switch1 : Switch  Criteria=u2 ~= 0  Threshold=double(0)  OutDataTypeStr=int16  SampleTime=1e-08  SaturateOnIntegerOverflow=off  InputSameDT=off
  Resett_switch2 : Switch  Criteria=u2 ~= 0  Threshold=double(0)  OutDataTypeStr=int16  SampleTime=1e-08  SaturateOnIntegerOverflow=off  InputSameDT=off
  rd_{0..6} (7 alike) : Delay  DelayLength=double(1)  InitialCondition=0  SampleTime=1e-08
  reset_old_switch1 : Switch  Criteria=u2 ~= 0  Threshold=double(0)  OutDataTypeStr=int16  SampleTime=1e-08  SaturateOnIntegerOverflow=off  InputSameDT=off
  speed_old_switch1 : Switch  Criteria=u2 ~= 0  Threshold=double(0)  OutDataTypeStr=int16  SampleTime=1e-08  SaturateOnIntegerOverflow=off  InputSameDT=off
  count : Outport  SampleTime=1e-08  VectorParamsAs1DForOutWhenUnconnected=off
  wires:
  rd_2/1 -> Resett_switch2/2, reset_old_switch1/2
  Reset/1 -> rd_2/1
  rd_5/1 -> Resett_switch1/2
  rd_1/1 -> Relational Operator/2
  rd_4/1 -> Resett_switch1/3
  rd_6/1 -> reset_old_switch1/3
  rd_3/1 -> speed_old_switch1/1
  rd_0/1 -> Reset_when_overflow/2
  Resett_switch1/1 -> reset_old_switch1/1, Relational Operator/1, Add1/2
  Relational Operator/1 -> rd_5/1
  Add1/1 -> Resett_switch2/3
  Resett_switch2/1 -> rd_4/1
  speed_old_switch1/1 -> Add1/1
  reset_old_switch1/1 -> count/1, rd_6/1
  Reset_when_overflow/1 -> rd_1/1
  Constant4/1 -> Reset_when_overflow/1
  Constant3/1 -> speed_old_switch1/3
  Constant2/1 -> rd_3/1
  Constant1/1 -> Resett_switch2/1, Resett_switch1/1
  IncsPerTurn/1 -> rd_0/1
  Edge/1 -> speed_old_switch1/2

== system gm_inc_enc_v26_vnl/IncEnc_V26/digital_filter ==
  A : Inport  OutDataTypeStr=boolean  PortDimensions=1  SampleTime=1e-08
  AND : Logic  Inputs=3  AllPortsSameDT=off  OutDataTypeStr=boolean  SampleTime=1e-08
  AND1 : Logic  Inputs=3  AllPortsSameDT=off  OutDataTypeStr=boolean  SampleTime=1e-08
  NOT : Logic  Operator=NOT  Inputs=1  AllPortsSameDT=off  OutDataTypeStr=boolean  SampleTime=1e-08
  NOT1 : Logic  Operator=NOT  Inputs=1  AllPortsSameDT=off  OutDataTypeStr=boolean  SampleTime=1e-08
  NOT2 : Logic  Operator=NOT  Inputs=1  AllPortsSameDT=off  OutDataTypeStr=boolean  SampleTime=1e-08
  Subsystem1 : Subsystem
  rd_0 : Delay  DelayLength=double(2)  InitialCondition=0  SampleTime=1e-08
  rd_{1..4} (4 alike) : Delay  DelayLength=double(1)  InitialCondition=0  SampleTime=1e-08
  Q : Outport  SampleTime=1e-08
  wires:
  rd_4/1 -> NOT2/1
  rd_2/1 -> rd_4/1, NOT1/1, AND/3
  rd_1/1 -> rd_2/1, NOT/1, AND/2
  rd_0/1 -> rd_1/1, AND/1
  A/1 -> rd_0/1
  rd_3/1 -> Subsystem1/1(S)
  Subsystem1/1(Q) -> Q/1
  NOT2/1 -> AND1/3
  NOT1/1 -> AND1/2
  NOT/1 -> AND1/1
  AND1/1 -> Subsystem1/2(R)
  AND/1 -> rd_3/1

== system gm_inc_enc_v26_vnl/IncEnc_V26/digital_filter1 ==
  A : Inport  OutDataTypeStr=boolean  PortDimensions=1  SampleTime=1e-08
  AND : Logic  Inputs=3  AllPortsSameDT=off  OutDataTypeStr=boolean  SampleTime=1e-08
  AND1 : Logic  Inputs=3  AllPortsSameDT=off  OutDataTypeStr=boolean  SampleTime=1e-08
  NOT : Logic  Operator=NOT  Inputs=1  AllPortsSameDT=off  OutDataTypeStr=boolean  SampleTime=1e-08
  NOT1 : Logic  Operator=NOT  Inputs=1  AllPortsSameDT=off  OutDataTypeStr=boolean  SampleTime=1e-08
  NOT2 : Logic  Operator=NOT  Inputs=1  AllPortsSameDT=off  OutDataTypeStr=boolean  SampleTime=1e-08
  Subsystem1 : Subsystem
  rd_0 : Delay  DelayLength=double(2)  InitialCondition=0  SampleTime=1e-08
  rd_{1..4} (4 alike) : Delay  DelayLength=double(1)  InitialCondition=0  SampleTime=1e-08
  Q : Outport  SampleTime=1e-08
  wires:
  rd_4/1 -> NOT2/1
  rd_2/1 -> rd_4/1, NOT1/1, AND/3
  rd_1/1 -> rd_2/1, NOT/1, AND/2
  rd_0/1 -> rd_1/1, AND/1
  A/1 -> rd_0/1
  rd_3/1 -> Subsystem1/1(S)
  Subsystem1/1(Q) -> Q/1
  NOT2/1 -> AND1/3
  NOT1/1 -> AND1/2
  NOT/1 -> AND1/1
  AND1/1 -> Subsystem1/2(R)
  AND/1 -> rd_3/1

== system gm_inc_enc_v26_vnl/IncEnc_V26/digital_filter2 ==
  A : Inport  OutDataTypeStr=boolean  PortDimensions=1  SampleTime=1e-08
  AND : Logic  Inputs=3  AllPortsSameDT=off  OutDataTypeStr=boolean  SampleTime=1e-08
  AND1 : Logic  Inputs=3  AllPortsSameDT=off  OutDataTypeStr=boolean  SampleTime=1e-08
  NOT : Logic  Operator=NOT  Inputs=1  AllPortsSameDT=off  OutDataTypeStr=boolean  SampleTime=1e-08
  NOT1 : Logic  Operator=NOT  Inputs=1  AllPortsSameDT=off  OutDataTypeStr=boolean  SampleTime=1e-08
  NOT2 : Logic  Operator=NOT  Inputs=1  AllPortsSameDT=off  OutDataTypeStr=boolean  SampleTime=1e-08
  Subsystem1 : Subsystem
  rd_0 : Delay  DelayLength=double(2)  InitialCondition=0  SampleTime=1e-08
  rd_{1..4} (4 alike) : Delay  DelayLength=double(1)  InitialCondition=0  SampleTime=1e-08
  Q : Outport  SampleTime=1e-08
  wires:
  rd_4/1 -> NOT2/1
  rd_2/1 -> rd_4/1, NOT1/1, AND/3
  rd_1/1 -> rd_2/1, NOT/1, AND/2
  rd_0/1 -> rd_1/1, AND/1
  A/1 -> rd_0/1
  rd_3/1 -> Subsystem1/1(S)
  Subsystem1/1(Q) -> Q/1
  NOT2/1 -> AND1/3
  NOT1/1 -> AND1/2
  NOT/1 -> AND1/1
  AND1/1 -> Subsystem1/2(R)
  AND/1 -> rd_3/1

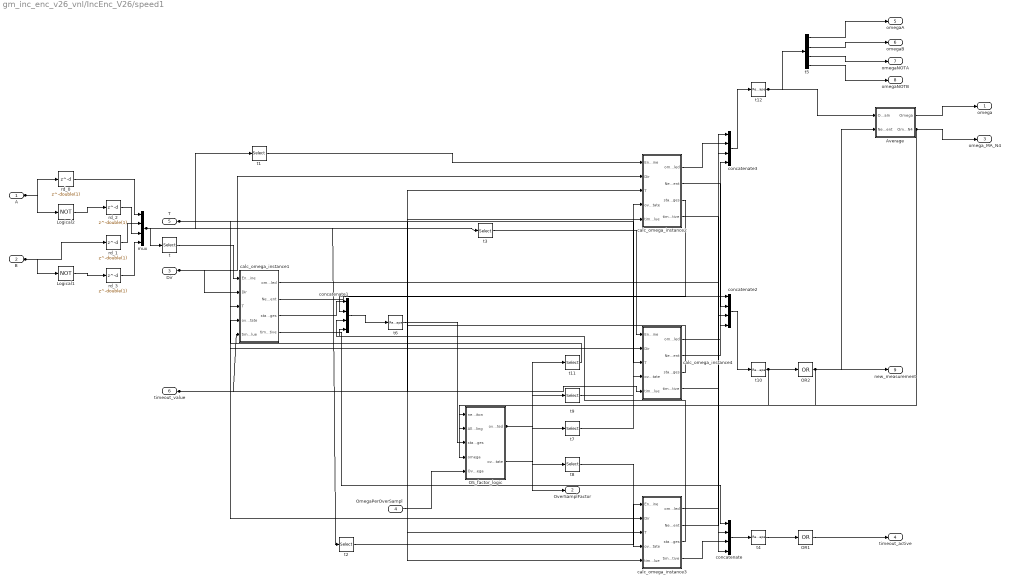
== system gm_inc_enc_v26_vnl/IncEnc_V26/speed1 ==
  A : Inport  OutDataTypeStr=boolean  PortDimensions=1  SampleTime=1e-08
  B : Inport  Port=2  OutDataTypeStr=boolean  PortDimensions=1  SampleTime=1e-08
  Dir : Inport  Port=3  OutDataTypeStr=fixdt(1, 4, 0)  PortDimensions=1  SampleTime=1e-08
  OmegaPerOverSampl : Inport  Port=4  OutDataTypeStr=fixdt(1, 24, 11)  PortDimensions=1  SampleTime=1e-08
  T : Inport  Port=5  OutDataTypeStr=fixdt(1, 38, 32)  PortDimensions=1  SampleTime=1e-08
  timeout_value : Inport  Port=6  OutDataTypeStr=uint32  PortDimensions=1  SampleTime=1e-08
  Average : Subsystem
  Logical1 : Logic  Operator=NOT  Inputs=1  AllPortsSameDT=off  OutDataTypeStr=boolean  SampleTime=1e-08
  Logical2 : Logic  Operator=NOT  Inputs=1  AllPortsSameDT=off  OutDataTypeStr=boolean  SampleTime=1e-08
  OR1 : Logic  Operator=OR  Inputs=1  AllPortsSameDT=off  OutDataTypeStr=boolean  SampleTime=1e-08
  OR2 : Logic  Operator=OR  Inputs=1  AllPortsSameDT=off  OutDataTypeStr=boolean  SampleTime=1e-08
  OS_factor_logic : Subsystem
  calc_omega_instance1 : Subsystem
  calc_omega_instance2 : Subsystem
  calc_omega_instance3 : Subsystem
  calc_omega_instance4 : Subsystem
  concatenate{,1..3} (4 alike) : Concatenate  NumInputs=4
  mux : Mux
  rd_{0..3} (4 alike) : Delay  DelayLength=double(1)  InitialCondition=0  SampleTime=1e-08
  t : Selector  SampleTime=1e-08  IndexOptions=Index vector (dialog)  Indices=double(1)  OutputSizes=1
  t1 : Selector  SampleTime=1e-08  IndexOptions=Index vector (dialog)  Indices=double(2)  OutputSizes=1
  t{4,6,10,12} (4 alike) : Reshape
  t11 : Selector  SampleTime=1e-08  IndexOptions=Index vector (dialog)  Indices=double(1)  OutputSizes=1
  t2 : Selector  SampleTime=1e-08  IndexOptions=Index vector (dialog)  Indices=double(3)  OutputSizes=1
  t3 : Selector  SampleTime=1e-08  IndexOptions=Index vector (dialog)  Indices=double(4)  OutputSizes=1
  t5 : Demux
  t7 : Selector  SampleTime=1e-08  IndexOptions=Index vector (dialog)  Indices=double(4)  OutputSizes=1
  t8 : Selector  SampleTime=1e-08  IndexOptions=Index vector (dialog)  Indices=double(3)  OutputSizes=1
  t9 : Selector  SampleTime=1e-08  IndexOptions=Index vector (dialog)  Indices=double(2)  OutputSizes=1
  omega : Outport  SampleTime=1e-08  VectorParamsAs1DForOutWhenUnconnected=off
  OverSamplFactor : Outport  Port=2  SampleTime=1e-08
  omega_MA_N4 : Outport  Port=3  SampleTime=1e-08  VectorParamsAs1DForOutWhenUnconnected=off
  timeout_active : Outport  Port=4  OutDataTypeStr=boolean  SampleTime=1e-08  VectorParamsAs1DForOutWhenUnconnected=off
  omegaA : Outport  Port=5  SampleTime=1e-08  VectorParamsAs1DForOutWhenUnconnected=off
  omegaB : Outport  Port=6  SampleTime=1e-08  VectorParamsAs1DForOutWhenUnconnected=off
  omegaNOTA : Outport  Port=7  SampleTime=1e-08  VectorParamsAs1DForOutWhenUnconnected=off
  omegaNOTB : Outport  Port=8  SampleTime=1e-08  VectorParamsAs1DForOutWhenUnconnected=off
  new_measurement : Outport  Port=9  OutDataTypeStr=boolean  SampleTime=1e-08  VectorParamsAs1DForOutWhenUnconnected=off
  wires:
  rd_2/1 -> mux/3
  rd_0/1 -> mux/1
  rd_3/1 -> mux/4
  rd_1/1 -> mux/2
  concatenate3/1 -> t12/1
  calc_omega_instance1/3(state_count_edges) -> concatenate1/1
  calc_omega_instance1/2(NewMeasurement) -> concatenate2/1
  calc_omega_instance1/1(omega_oversampled) -> concatenate3/1
  t11/1 -> calc_omega_instance1/4(oversampling_state)
  OS_factor_logic/1(oversampling_adjusted) -> t11/1, t9/1, t8/1, t7/1
  t10/1 -> OS_factor_logic/1(new_transisiton), OR2/1
  concatenate2/1 -> t10/1
  calc_omega_instance2/3(state_count_edges) -> concatenate1/2
  calc_omega_instance2/2(NewMeasurement) -> concatenate2/2
  calc_omega_instance2/1(omega_oversampled) -> concatenate3/2
  t9/1 -> calc_omega_instance2/4(oversampling_state)
  calc_omega_instance3/3(state_count_edges) -> concatenate1/3
  calc_omega_instance3/2(NewMeasurement) -> concatenate2/3
  calc_omega_instance3/1(omega_oversampled) -> concatenate3/3
  t8/1 -> calc_omega_instance3/4(oversampling_state)
  calc_omega_instance4/3(state_count_edges) -> concatenate1/4
  calc_omega_instance4/2(NewMeasurement) -> concatenate2/4
  calc_omega_instance4/1(omega_oversampled) -> concatenate3/4
  t7/1 -> calc_omega_instance4/4(oversampling_state)
  t6/1 -> OS_factor_logic/3(state_edges)
  concatenate1/1 -> t6/1
  t5/4 -> omegaNOTB/1
  t5/3 -> omegaNOTA/1
  t5/2 -> omegaB/1
  t5/1 -> omegaA/1
  calc_omega_instance4/4(timeout_active) -> concatenate/4
  calc_omega_instance3/4(timeout_active) -> concatenate/3
  calc_omega_instance2/4(timeout_active) -> concatenate/2
  calc_omega_instance1/4(timeout_active) -> concatenate/1
  concatenate/1 -> t4/1
  t3/1 -> calc_omega_instance4/1(Encoder Line)
  t2/1 -> calc_omega_instance3/1(Encoder Line)
  t1/1 -> calc_omega_instance2/1(Encoder Line)
  t/1 -> calc_omega_instance1/1(Encoder Line)
  t4/1 -> OR1/1
  t12/1 -> Average/1("OmegaIn "), t5/1
  OS_factor_logic/2(oversampling_state) -> OverSamplFactor/1
  OR2/1 -> OS_factor_logic/2(Allow_ToCheckOversampling), Average/2(NewMeasurement), new_measurement/1
  OR1/1 -> timeout_active/1
  mux/1 -> t/1, t1/1, t2/1, t3/1
  Logical2/1 -> rd_2/1
  Logical1/1 -> rd_3/1
  Average/2(OmegaOut_MA_N4) -> OS_factor_logic/4(omega), omega_MA_N4/1
  Average/1(Omega) -> omega/1
  timeout_value/1 -> calc_omega_instance4/5(timeout_value), calc_omega_instance3/5(timeout_value), calc_omega_instance2/5(timeout_value), calc_omega_instance1/5(timeout_value)
  T/1 -> calc_omega_instance4/3(T), calc_omega_instance3/3(T), calc_omega_instance2/3(T), calc_omega_instance1/3(T)
  OmegaPerOverSampl/1 -> OS_factor_logic/5(OverSamplOmega)
  Dir/1 -> calc_omega_instance4/2(Dir), calc_omega_instance3/2(Dir), calc_omega_instance2/2(Dir), calc_omega_instance1/2(Dir)
  B/1 -> Logical1/1, rd_1/1
  A/1 -> Logical2/1, rd_0/1

== system gm_inc_enc_v26_vnl/IncEnc_V26_vnl/AB-Line-Switch ==
  A_in : Inport
  B_in : Inport  Port=2
  CW_CCW_Switch : Inport  Port=3
  Switch : Switch  Criteria=u2 > Threshold  SaturateOnIntegerOverflow=off  InputSameDT=off
  Switch1 : Switch  Criteria=u2 > Threshold  SaturateOnIntegerOverflow=off  InputSameDT=off
  A_out : Outport
  B_out : Outport  Port=2
  wires:
  CW_CCW_Switch/1 -> Switch/2, Switch1/2
  A_in/1 -> Switch/3, Switch1/1
  B_in/1 -> Switch1/3, Switch/1
  Switch1/1 -> B_out/1
  Switch/1 -> A_out/1
